simulink model "DynamicModel"  (R2019a)
settings: Solver=VariableStepAuto  StartTime=0.0  StopTime=10.0  RelTol=1e-3
libraries: fl_lib x7, nesl_utility x6, ee_lib x1
settings Model: Creator=nikos  LastModifiedBy=nikos

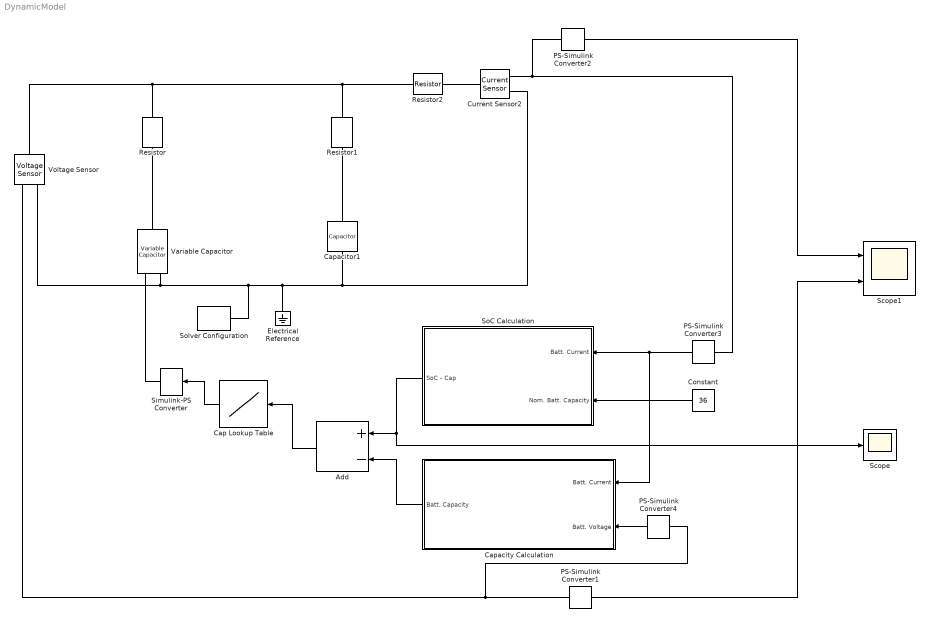
== system DynamicModel ==
  Add : Sum  Inputs=+-
  Cap Lookup Table : Lookup_n-D  NumberOfTableDimensions=1  BreakpointsForDimension1=[0,10,20,30,40,50,60,70,80,90,100]  Table=[1.4743,1.6265,2.2758,1.9491,2.3622,1.7126,1.7612,1.9919,1.4049,1.6798,1.4178]  InternalRulePriority=Speed  RndMeth=Simplest  InputSameDT=on
  Capacitor1 : fl_lib/Electrical/Electrical Elements/Capacitor  c=0.5 F  r=1e-6 Ohm  g=0 1/Ohm  i_specify=off  i_priority=High  i=0 A  i_nominal_specify=off  i_nominal_unit=A  i_nominal_value=1  v_specify=off  v_priority=High  v=0 V  v_nominal_specify=off  v_nominal_unit=V  v_nominal_value=1  vc_specify=off  vc_priority=High  vc=0 V  vc_nominal_specify=off  vc_nominal_unit=V  vc_nominal_value=1
  Capacity Calculation : Subsystem
  Constant : Constant  Value=36
  Current Sensor2 : fl_lib/Electrical/Electrical Sensors/Current Sensor
  Electrical Reference : fl_lib/Electrical/Electrical Elements/Electrical Reference
  PS-Simulink Converter{1..4} (4 alike) : nesl_utility/PS-Simulink Converter  PhysicalDomain=network_engine_domain  SubClassName=ps_output  LeftPortType=input  RightPortType=output  PseudoPeriodic=off  Frequencies=[]  Unit=1  AffineConversion=off
  Resistor : fl_lib/Electrical/Electrical Elements/Resistor  R=0.5 Ohm  i_specify=off  i_priority=High  i=0 A  i_nominal_specify=off  i_nominal_unit=A  i_nominal_value=1  v_specify=off  v_priority=High  v=0 V  v_nominal_specify=off  v_nominal_unit=V  v_nominal_value=1
  Resistor1 : fl_lib/Electrical/Electrical Elements/Resistor  R=1.5 Ohm  i_specify=off  i_priority=High  i=0 A  i_nominal_specify=off  i_nominal_unit=A  i_nominal_value=1  v_specify=off  v_priority=High  v=0 V  v_nominal_specify=off  v_nominal_unit=V  v_nominal_value=1
  Resistor2 : fl_lib/Electrical/Electrical Elements/Resistor  R=0.5 Ohm  i_specify=off  i_priority=High  i=0 A  i_nominal_specify=off  i_nominal_unit=A  i_nominal_value=1  v_specify=off  v_priority=High  v=0 V  v_nominal_specify=off  v_nominal_unit=V  v_nominal_value=1
  Scope : Scope
  Scope1 : Scope  NumInputPorts=2
  Simulink-PS Converter : nesl_utility/Simulink-PS Converter  PhysicalDomain=network_engine_domain  SubClassName=ps_input  LeftPortType=input  RightPortType=output  PseudoPeriodic=off  Frequencies=[]  NoiseDistribution=none  NoiseParameters=[]  Unit=1  AffineConversion=off  FilteringAndDerivatives=zero  SimscapeFilterOrder=1  InputFilterTimeConstant=0.001  UdotUserProvided=1
  SoC Calculation : Subsystem
  Solver Configuration : nesl_utility/Solver Configuration  PhysicalDomain=network_engine_domain  SubClassName=solver  LeftPortType=input  RightPortType=generic  Tones=[]  Harmonics=[]  SimulateNoise=off  Profile=off  UseLocalSampling=off  EnableSwitchedLinearOptims=on  FrequencyDomain=off  UseCCode=off  RelTol=0.001  AbsTol=1e-06  MinStep=1e-09  ToWorkspace=off  RevertToSquareIcSolve=off  NumHomotopyIterations=100  PhasorMode=off  PhasorModeNumHarmonics=1  DoDC=off  ResidualTolerance=1e-09  UseLocalSolver=off  LocalSolverChoice=NE_BACKWARD_EULER_ADVANCER  LocalSolverSampleTime=0.001  DoFixedCost=off  MaxNonlinIter=3  MaxModeIter=2  LinearAlgebra=Sparse  EquationFormulation=NE_TIME_EF  DelaysMemoryBudget=1024  AutomaticFiltering=on  FilteringTimeConstant=0.001  PartitionStorageMethod=AS_NEEDED  PartitionMemoryBudget=1024  PartitionMethod=FAST
  Variable Capacitor : ee_lib/Passive/Variable Capacitor  prm=2  Cmin=1 F  r=1e-6 Ohm  v0=0 V  q0=0 c
      settings: SourceProductName=Simscape Electrical  SourceProductBaseCode=PS
  Voltage Sensor : fl_lib/Electrical/Electrical Sensors/Voltage Sensor
  wires:
  Constant/1 -> SoC Calculation/2("Nom. Batt. Capacity ")
  PS-Simulink Converter3/1 -> Capacity Calculation/1(Batt. Current), SoC Calculation/1("Batt. Current ")
  Cap Lookup Table/1 -> Simulink-PS Converter/1
  PS-Simulink Converter2/1 -> Scope1/1
  PS-Simulink Converter1/1 -> Scope1/2
  PS-Simulink Converter4/1 -> Capacity Calculation/2("Batt. Voltage ")
  SoC Calculation/1(SoC - Cap) -> Scope/1, Add/1
  Capacity Calculation/1("Batt. Capacity ") -> Add/2
  Add/1 -> Cap Lookup Table/1
  connections:
  Resistor1/RConn1 -- Resistor2/LConn1 -- Resistor/RConn1 -- Voltage Sensor/LConn1
  Current Sensor2/RConn1 -- PS-Simulink Converter3/LConn1 -- PS-Simulink Converter2/LConn1
  Current Sensor2/LConn1 -- Resistor2/RConn1
  Simulink-PS Converter/RConn1 -- Variable Capacitor/LConn1
  Variable Capacitor/RConn1 -- Resistor/LConn1
  Capacitor1/LConn1 -- Current Sensor2/RConn2 -- Electrical Reference/LConn1 -- Solver Configuration/RConn1 -- Variable Capacitor/LConn2 -- Voltage Sensor/RConn2
  PS-Simulink Converter1/LConn1 -- PS-Simulink Converter4/LConn1 -- Voltage Sensor/RConn1
  Capacitor1/RConn1 -- Resistor1/LConn1

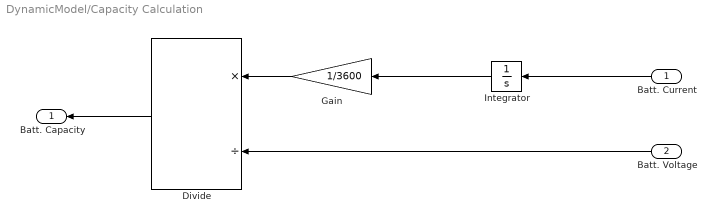
== system DynamicModel/Capacity Calculation ==
  Batt. Current : Inport
  "Batt. Voltage " : Inport  Port=2
  Divide : Product  Inputs=*/
  Gain : Gain  Gain=1/3600
  Integrator : Integrator
  "Batt. Capacity " : Outport
  wires:
  Batt. Current/1 -> Integrator/1
  Integrator/1 -> Gain/1
  "Batt. Voltage "/1 -> Divide/2
  Gain/1 -> Divide/1
  Divide/1 -> "Batt. Capacity "/1

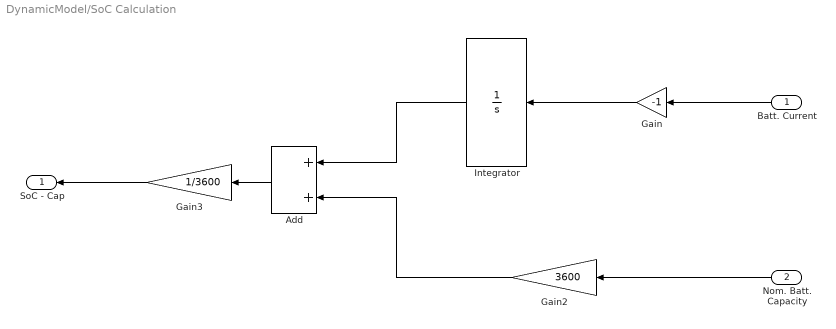
== system DynamicModel/SoC Calculation ==
  "Batt. Current " : Inport
  "Nom. Batt. Capacity " : Inport  Port=2  OutMin=0  OutMax=100
  Add : Sum
  Gain : Gain  Gain=-1
  Gain2 : Gain  Gain=3600
  Gain3 : Gain  Gain=1/3600
  Integrator : Integrator
  SoC - Cap : Outport
  wires:
  "Batt. Current "/1 -> Gain/1
  Gain/1 -> Integrator/1
  "Nom. Batt. Capacity "/1 -> Gain2/1
  Gain2/1 -> Add/2
  Add/1 -> Gain3/1
  Integrator/1 -> Add/1
  Gain3/1 -> SoC - Cap/1
